simulink model "torque_pi_controller"  (R2023b)
settings: Solver=VariableStepAuto  StartTime=0.0  StopTime=10.0  RelTol=1e-5
values from neighbouring files (symbols this model uses):
  K = 1.339    [torque_PI_integral_algorithm.m]    (also in torque_PI_tuning.m; torque_model.m = 1.32)
libraries: cstblocks x1
settings Model: Creator=paoli  LastModifiedBy=kiraa

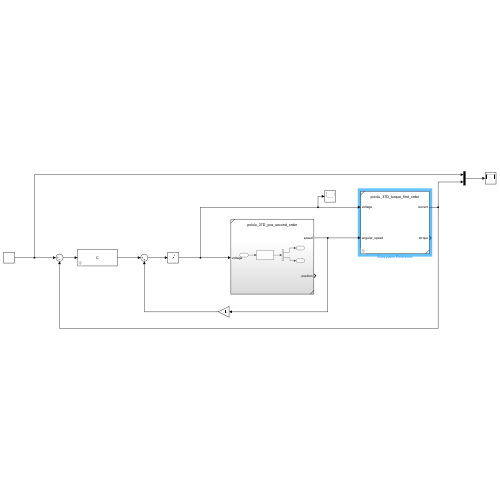
[thumbnail: Simulink's stored preview of the top-level diagram]
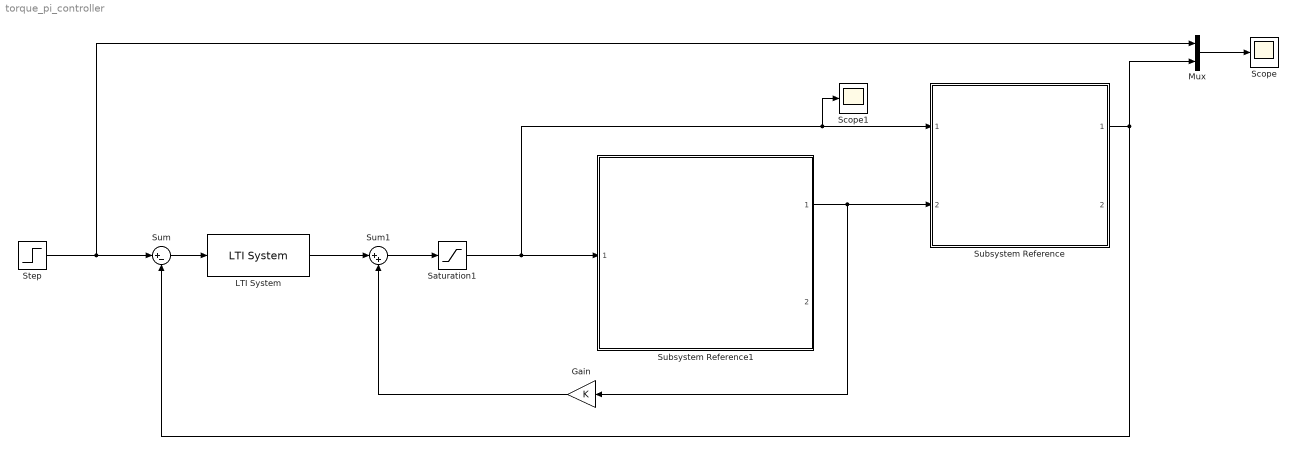
== system torque_pi_controller ==
  Gain : Gain  Gain=K
  LTI System : cstblocks/LTI System  sys=C  IC=[]  PadeOrder=0
  Mux : Mux  Inputs=2
  Saturation1 : Saturate  UpperLimit=12  LowerLimit=-12
  Scope : Scope
  Scope1 : Scope
  Step : Step  Time=3  Before=1  After=0  SampleTime=0
  Subsystem Reference : Subsystem  ReferencedSubsystem=pololu_37D_torque_first_order  L=2.3e-3  R=1.7  K=1.339
  Subsystem Reference1 : Subsystem  ReferencedSubsystem=pololu_37D_pos_second_order
  Sum : Sum  Inputs=|+-
  Sum1 : Sum  Inputs=|++
  wires:
  Subsystem Reference/1 -> Sum/2, Mux/2
  Sum/1 -> LTI System/1
  Step/1 -> Mux/1, Sum/1
  Mux/1 -> Scope/1
  Subsystem Reference1/1 -> Subsystem Reference/2, Gain/1
  Sum1/1 -> Saturation1/1
  LTI System/1 -> Sum1/1
  Gain/1 -> Sum1/2
  Saturation1/1 -> Scope1/1, Subsystem Reference/1, Subsystem Reference1/1
